simulink model "opticalflow"  (Simulink 7.1)
settings: Solver=ode45  StartTime=0.0  StopTime=10.0  RelTol=1e-3
undefined symbols (not defined in the file or in its folder): gray, Horn, Rec, Schunck, SDTV
libraries: vipsnks x3, vipconversions x1, viptextngfix x1, dspsrcs4 x1, vipanalysis x1, dspsnks4 x1
settings Model: Creator=stevenw  LastModifiedBy=stevenw

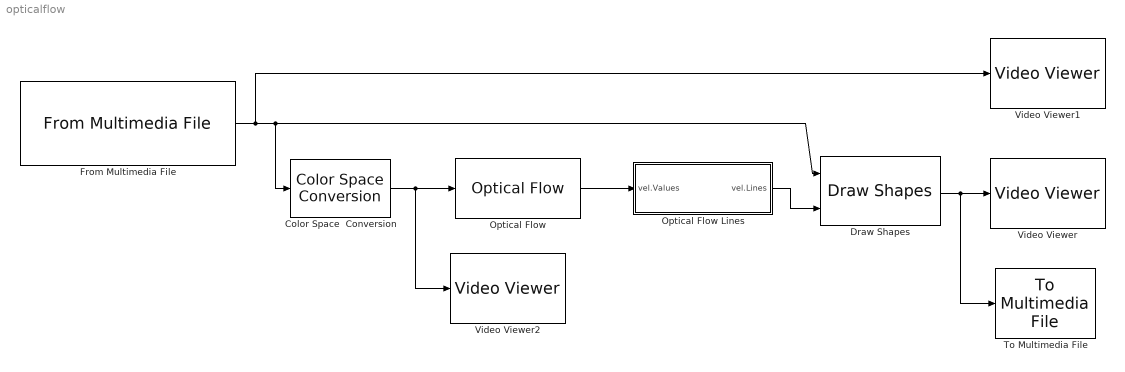
== system opticalflow ==
  Color Space  Conversion : vipconversions/Color Space  Conversion  conversion=Obsolete  conversionActive=R'G'B' to intensity  wp_str=D65  rec=Rec. 601 (SDTV)  sys=1125/60/2:1  imagePorts=One multidimensional signal
  Draw Shapes : viptextngfix/Draw Shapes  DialogController=vipDDGCreate  DialogControllerArgs=DataTag0  shape=Lines  fill=off  display=User-specified value  intensity=200  color=[255 255 0]  opacity=0.6  viewport=Entire image  antialiasing=off  inType=Obsolete  imagePorts=One multidimensional signal
  From Multimedia File : dspsrcs4/From Multimedia File  DialogController=dspDDGCreate  DialogControllerArgs=DataTag1  inputFilename=trafficlanes.avi  loop=on  numPlays=inf  outputStreams=Video only  videoDataType=single  audioDataType=int16  inheritSampleTime=on  userDefinedSampleTime=1/30  noAudioOutput=off  isIntensityVideo=off  colorVideoFormat=One multidimensional signal  outputEOF=off  dataOrg=Column-major
  Optical Flow : vipanalysis/Optical Flow  DialogController=vipDDGCreate  DialogControllerArgs=DataTag2  SystemSampleTime=-1  method=Horn-Schunck  gradMethod=Difference filter [-1 1]  which2img=Current frame and N-th frame back  N=1  outVelForm=Horizontal and vertical components in complex form  lambda=1  stop_criteria=When maximum number of iterations is reached  maxAllowAbsDiff=eps  maxIter=10  numInports=3  sigmaS=1.5  sigmaW=1  eigTh=0.0039  discardNormalFlow=off  outputCurrentImage=off  prodOutputMode=Binary point scaling  prodOutputWordLength=32  prodOutputFracLength=20  outputMode=Binary point scaling  outputWordLength=32  outputFracLength=20  roundingMode=Nearest  overflowMode=on
  Optical Flow Lines : Subsystem  mask(Optical Flow Lines){scaleFactor=40}
      mask prompts: scaleFactor "Motion vector gain:"
      mask help: Generates the coordinate points of optical flow lines.
      mask Help: Generates the coordinate points of optical flow lines. Look under its mask to see the implementation details.
  To Multimedia File : dspsnks4/To Multimedia File  DialogController=dspDDGCreate  DialogControllerArgs=DataTag3  outputFilename=flow.avi  streamSelection=Video only  videoCompressor=None (uncompressed)  audioCompressor=None (uncompressed)  imagePorts=One multidimensional signal
  Video Viewer : vipsnks/Video Viewer  DialogController=vipDDGCreate  DialogControllerArgs=DataTag4  inputType=Obsolete7b  imagePorts=One multidimensional signal  useColorMap=off  colormapValue=gray(256)  specRange=off  minInputVal=0  maxInputVal=255  FigPos=[780 473 360 240]  AxisZoom=on  trueSizedOnce=on
  Video Viewer1 : vipsnks/Video Viewer  DialogController=vipDDGCreate  DialogControllerArgs=DataTag5  inputType=Obsolete7b  imagePorts=One multidimensional signal  useColorMap=off  colormapValue=gray(256)  specRange=off  minInputVal=0  maxInputVal=255  FigPos=[780 473 360 240]  AxisZoom=on  trueSizedOnce=on
  Video Viewer2 : vipsnks/Video Viewer  DialogController=vipDDGCreate  DialogControllerArgs=DataTag6  inputType=Obsolete7b  imagePorts=One multidimensional signal  useColorMap=off  colormapValue=gray(256)  specRange=off  minInputVal=0  maxInputVal=255  FigPos=[780 473 360 240]  AxisZoom=on  trueSizedOnce=on
  wires:
  From Multimedia File/1 -> Color Space  Conversion/1, Draw Shapes/1, Video Viewer1/1
  Color Space  Conversion/1 -> Optical Flow/1, Video Viewer2/1
  Optical Flow/1 -> Optical Flow Lines/1(vel.Values)
  Optical Flow Lines/1(vel.Lines) -> Draw Shapes/2
  Draw Shapes/1 -> Video Viewer/1, To Multimedia File/1

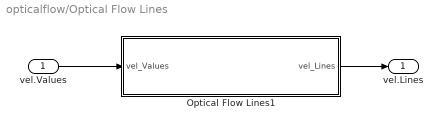
== system opticalflow/Optical Flow Lines ==
  vel.Values : Inport  OutDataType=sfix(16)  OutScaling=2^0
  Optical Flow Lines1 : Stateflow chart
  vel.Lines : Outport  OutDataType=sfix(16)  OutScaling=2^0
  wires:
  vel.Values/1 -> Optical Flow Lines1/1(vel_Values)
  Optical Flow Lines1/1(vel_Lines) -> vel.Lines/1

== matlab function Optical Flow Lines/Optical Flow Lines1 ==
  data: vel_Values input double; vel_Lines output double; scaleFactor parameter double size=1
function vel_Lines=OpticalFlowLines(vel_Values, scaleFactor) 

% Generates the coordinate points of optical flow lines

persistent first_time;
persistent X;
persistent Y;
persistent RV;
persistent CV;
if isempty(first_time)
    first_time     = 1;
    %% user may change the following three parameters
    borderOffset   = 5;
    decimFactorRow = 5;
    decimFactorCol = 5;    
    %%
    [R C] = size(vel_Values);
    RV = borderOffset:decimFactorRow:(R-borderOffset);   
    CV = borderOffset:decimFactorCol:(C-borderOffset);
    [Y X] = meshgrid(CV,RV);
end

tmp = vel_Values(RV,CV);
tmp = tmp.*scaleFactor;
vel_Lines = [X(:)';Y(:)';X(:)'+imag(tmp(:))';Y(:)'+real(tmp(:))'];
